simulink model "modelo"  (R2020a)
settings: Solver=VariableStepAuto  StartTime=0.0  StopTime=0.001  RelTol=1e-3
values from neighbouring files (symbols this model uses):
  C = 4    [ilaplace.m]    (also in laplaceEjercicioRLC.m = 0.1)
  L = 1    [ilaplace.m]    (also in laplaceEjercicioRLC.m = 0.5)
  R = 0    [ilaplace.m]    (also in laplaceEjercicioRLC.m = 1)
settings Model: Creator=personal  LastModifiedBy=personal

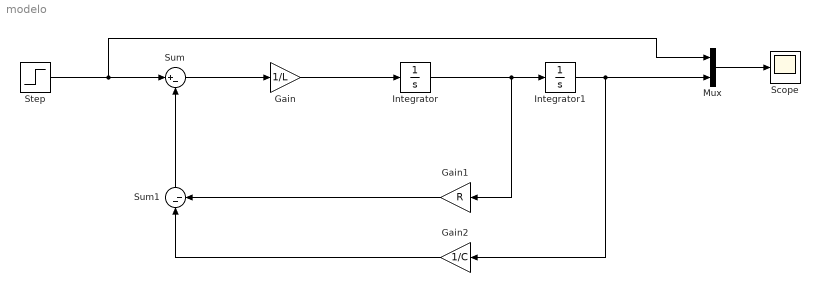
== system modelo ==
  Gain : Gain  Gain=1/L
  Gain1 : Gain  Gain=R
  Gain2 : Gain  Gain=1/C
  Integrator : Integrator
  Integrator1 : Integrator
  Mux : Mux  Inputs=2
  Scope : Scope
  Step : Step  Before=5  After=0  SampleTime=0
  Sum : Sum  Inputs=|+-
  Sum1 : Sum  Inputs=|--
  wires:
  Gain/1 -> Integrator/1
  Integrator/1 -> Gain1/1, Integrator1/1
  Sum/1 -> Gain/1
  Step/1 -> Mux/1, Sum/1
  Integrator1/1 -> Gain2/1, Mux/2
  Mux/1 -> Scope/1
  Gain1/1 -> Sum1/2
  Sum1/1 -> Sum/2
  Gain2/1 -> Sum1/1
